simulink model "simpleSmOffPSZ"  (Simulink 7.8)
settings: Solver=FixedStepDiscrete  StartTime=0.0  StopTime=inf  FixedStep=900  RelTol=1e-3
libraries: simulink x2
settings Model: Creator=mwetter  LastModifiedBy=wbernal  ExtModeAutoUpdateStatusClock=off
settings OptimizationCC: InitFltsAndDblsToZero=on
settings DebuggingCC: SaveWithParameterizedLinksMsg=none  FcnCallInpInsideContextMsg=Use local settings  StrictBusMsg=Warning
settings SFSimCC: SimParseCustomCode=off
settings GRTTargetCC: TargetFcnLib=ansi_tfl_tmw.mat

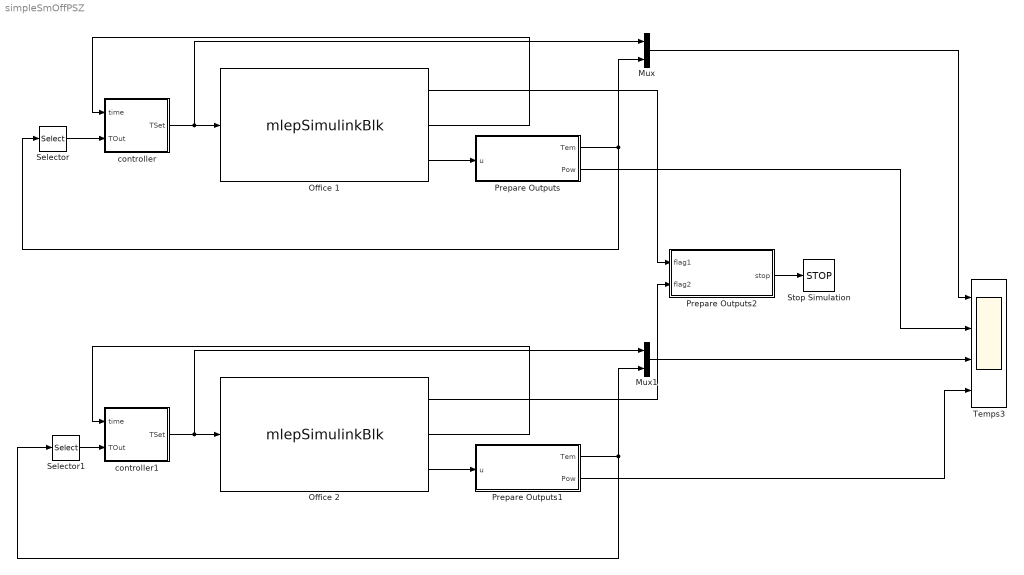
== system simpleSmOffPSZ ==
  Mux : Mux  Inputs=2
  Mux1 : Mux  Inputs=2
  Office 1 : M-S-Function  FunctionName=mlepSimulinkBlk  Parameters=progname, modelfile, weatherfile, workdir, timeout, port, host, bcvtbdir, deltaT, noutputd  mask(EnergyPlus Cosimulation){progname='C:\\EnergyPlusV8-0-0-mlep\\RunEPlus.bat', modelfile='U:\\Simulink-mlep\\SmOffPSZ1\\SmOffPSZ', weatherfile='USA_IL_Chicago-OHare.Intl.AP.725300_TMY3', workdir='U:\\Simulink-mlep\\SmOffPSZ1', timeout=2000, port=0, host='', bcvtbdir='U:\\Simulink-mlep\\bcvtb', deltaT=900, noutputd=14}
      mask prompts: progname "E+ Executable Path"; modelfile "IDF File (without extension)"; weatherfile "Weather Profile"; workdir "Working Directory"; timeout "Timeout (in milliseconds)"; port "Socket Port (0 = any available)"; host "Socket Host ('' = local host)"; bcvtbdir "BCVTB Directory"; deltaT "Time Step (in seconds)"; noutputd "Number of Real Outputs"
      mask help: This block implements cosimulation with EnergyPlus by allowing Simulink to exchange input and output data with it. Currently, EnergyPlus only supports real data.
      mask Help:
      | This block implements cosimulation with EnergyPlus by allowing Simulink to
      | exchange input and output data with it.
      | 
      | When a simulation starts, EnergyPlus is also started. It will then run in
      | parallel with Simulink. They exchange input and output data via socket
      | communication. When the simulation terminates, EnergyPlus will exit.
      | 
      | Refer to the manuals of MLE+ and/or BCVTB/EnergyPlus for details.
      | 
      | INPUTS:
      | - real: real vector input to EnergyPlus.
      | 
      | OUTPUTS:
      | - flag: status of EnergyPlus (0 if OK, if flag is non-zero, the simulation should stop).
      | - time: current simulation time of EnergyPlus, in seconds.
      | - real: real vector output from EnergyPlus.
      mask Display:
      | disp('E+\nCosimulation');
      | port_label('output', 1, 'flag');
      | port_label('output', 2, 'time');
      | port_label('output', 3, 'real');
      | % port_label('output', 4, 'int');
      | % port_label('output', 5, 'bool');
      | port_label('input', 1, 'real');
      | % port_label('input', 2, 'int');
      | % port_label('input', 3, 'bool');
      | image(imread('SmOffPSZ.png'))
  Office 2 : M-S-Function  FunctionName=mlepSimulinkBlk  Parameters=progname, modelfile, weatherfile, workdir, timeout, port, host, bcvtbdir, deltaT, noutputd  mask(EnergyPlus Cosimulation){progname='C:\\EnergyPlusV8-0-0-mlep\\RunEPlus.bat', modelfile='U:\\Simulink-mlep\\SmOffPSZ2\\SmOffPSZ', weatherfile='USA_IL_Chicago-OHare.Intl.AP.725300_TMY3', workdir='U:\\Simulink-mlep\\SmOffPSZ2', timeout=2000, port=0, host='', bcvtbdir='U:\\Simulink-mlep\\bcvtb', deltaT=900, noutputd=14}
      mask prompts: progname "E+ Executable Path"; modelfile "IDF File (without extension)"; weatherfile "Weather Profile"; workdir "Working Directory"; timeout "Timeout (in milliseconds)"; port "Socket Port (0 = any available)"; host "Socket Host ('' = local host)"; bcvtbdir "BCVTB Directory"; deltaT "Time Step (in seconds)"; noutputd "Number of Real Outputs"
      mask help: This block implements cosimulation with EnergyPlus by allowing Simulink to exchange input and output data with it. Currently, EnergyPlus only supports real data.
      mask Help:
      | This block implements cosimulation with EnergyPlus by allowing Simulink to
      | exchange input and output data with it.
      | 
      | When a simulation starts, EnergyPlus is also started. It will then run in
      | parallel with Simulink. They exchange input and output data via socket
      | communication. When the simulation terminates, EnergyPlus will exit.
      | 
      | Refer to the manuals of MLE+ and/or BCVTB/EnergyPlus for details.
      | 
      | INPUTS:
      | - real: real vector input to EnergyPlus.
      | 
      | OUTPUTS:
      | - flag: status of EnergyPlus (0 if OK, if flag is non-zero, the simulation should stop).
      | - time: current simulation time of EnergyPlus, in seconds.
      | - real: real vector output from EnergyPlus.
      mask Display:
      | disp('E+\nCosimulation');
      | port_label('output', 1, 'flag');
      | port_label('output', 2, 'time');
      | port_label('output', 3, 'real');
      | % port_label('output', 4, 'int');
      | % port_label('output', 5, 'bool');
      | port_label('input', 1, 'real');
      | % port_label('input', 2, 'int');
      | % port_label('input', 3, 'bool');
      | image(imread('SmOffPSZ.png'))
  Prepare Outputs : MATLAB Function  TreatAsAtomicUnit=on
  Prepare Outputs1 : MATLAB Function  TreatAsAtomicUnit=on
  Prepare Outputs2 : MATLAB Function  TreatAsAtomicUnit=on
  Selector : Selector  InputPortWidth=2  IndexOptions=Index vector (dialog)  Indices=[1]  OutputSizes=1
  Selector1 : Selector  InputPortWidth=2  IndexOptions=Index vector (dialog)  Indices=[1]  OutputSizes=1
  Stop Simulation : Stop
  Temps3 : Scope  NumInputPorts=4
      settings: YMin=-5~-5~-5~-5  YMax=5~5~5~5  SaveName=ScopeData3
  controller : Subsystem
  controller1 : Subsystem
  wires:
  controller/1(TSet) -> Mux/1, Office 1/1
  Office 1/2 -> controller/1(time)
  Mux/1 -> Temps3/1
  Selector/1 -> controller/2(TOut)
  Office 1/3 -> Prepare Outputs/1(u)
  Prepare Outputs/1(Tem) -> Mux/2, Selector/1
  Prepare Outputs/2(Pow) -> Temps3/2
  controller1/1(TSet) -> Mux1/1, Office 2/1
  Office 2/2 -> controller1/1(time)
  Mux1/1 -> Temps3/3
  Office 2/3 -> Prepare Outputs1/1(u)
  Prepare Outputs1/1(Tem) -> Mux1/2, Selector1/1
  Prepare Outputs1/2(Pow) -> Temps3/4
  Selector1/1 -> controller1/2(TOut)
  Prepare Outputs2/1(stop) -> Stop Simulation/1
  Office 1/1 -> Prepare Outputs2/1(flag1)
  Office 2/1 -> Prepare Outputs2/2(flag2)

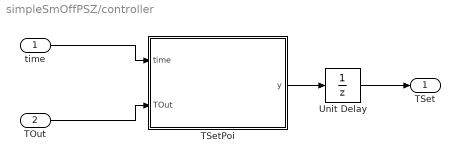
== system simpleSmOffPSZ/controller ==
  time : Inport
  TOut : Inport  Port=2
  TSetPoi : Subsystem
  Unit Delay : UnitDelay  X0=[20, 25]  SampleTime=-1
  TSet : Outport
  wires:
  time/1 -> TSetPoi/1(time)
  TOut/1 -> TSetPoi/2(TOut)
  Unit Delay/1 -> TSet/1
  TSetPoi/1(y) -> Unit Delay/1

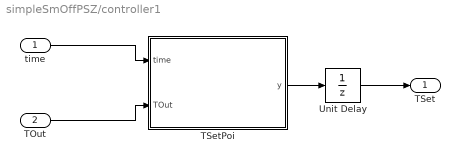
== system simpleSmOffPSZ/controller1 ==
  time : Inport
  TOut : Inport  Port=2
  TSetPoi : Subsystem
  Unit Delay : UnitDelay  X0=[20, 25]  SampleTime=-1
  TSet : Outport
  wires:
  time/1 -> TSetPoi/1(time)
  TOut/1 -> TSetPoi/2(TOut)
  Unit Delay/1 -> TSet/1
  TSetPoi/1(y) -> Unit Delay/1

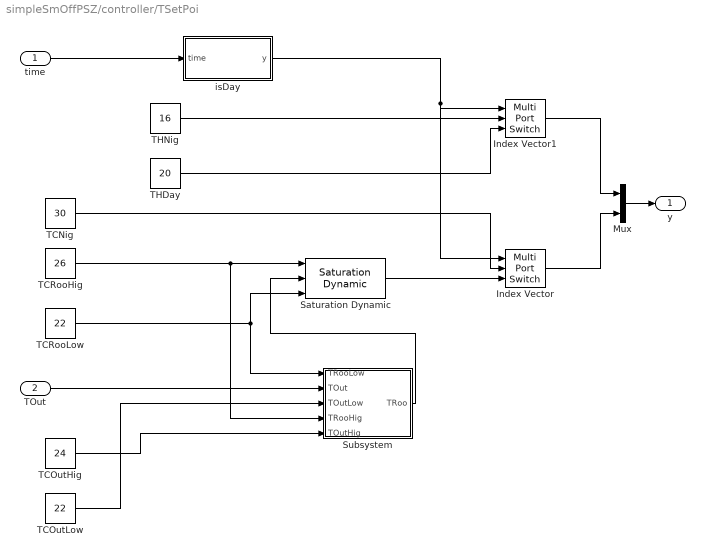
== system simpleSmOffPSZ/controller/TSetPoi ==
  time : Inport
  TOut : Inport  Port=2
  Index Vector : MultiPortSwitch  DataPortOrder=Zero-based contiguous  Inputs=2  zeroidx=on
  Index Vector1 : MultiPortSwitch  DataPortOrder=Zero-based contiguous  Inputs=2  zeroidx=on
  Mux : Mux  Inputs=2
  Saturation Dynamic : simulink/Discontinuities/Saturation Dynamic  OutMin=[]  OutMax=[]  OutDataTypeStr=Inherit: Same as second input  OutDataType=sfix(16)  OutScaling=2^-10  DoSatur=off
  Subsystem : Subsystem
  TCNig : Constant  Value=30
  TCOutHig : Constant  Value=24
  TCOutLow : Constant  Value=22
  TCRooHig : Constant  Value=26
  TCRooLow : Constant  Value=22
  THDay : Constant  Value=20
  THNig : Constant  Value=16
  isDay : Subsystem
  y : Outport
  wires:
  TOut/1 -> Subsystem/2(TOut)
  TCOutLow/1 -> Subsystem/3(TOutLow)
  TCOutHig/1 -> Subsystem/5(TOutHig)
  TCRooHig/1 -> Saturation Dynamic/1, Subsystem/4(TRooHig)
  TCRooLow/1 -> Saturation Dynamic/3, Subsystem/1(TRooLow)
  time/1 -> isDay/1(time)
  isDay/1(y) -> Index Vector/1, Index Vector1/1
  TCNig/1 -> Index Vector/2
  Subsystem/1(TRoo) -> Saturation Dynamic/2
  Saturation Dynamic/1 -> Index Vector/3
  THNig/1 -> Index Vector1/2
  THDay/1 -> Index Vector1/3
  Index Vector1/1 -> Mux/1
  Index Vector/1 -> Mux/2
  Mux/1 -> y/1

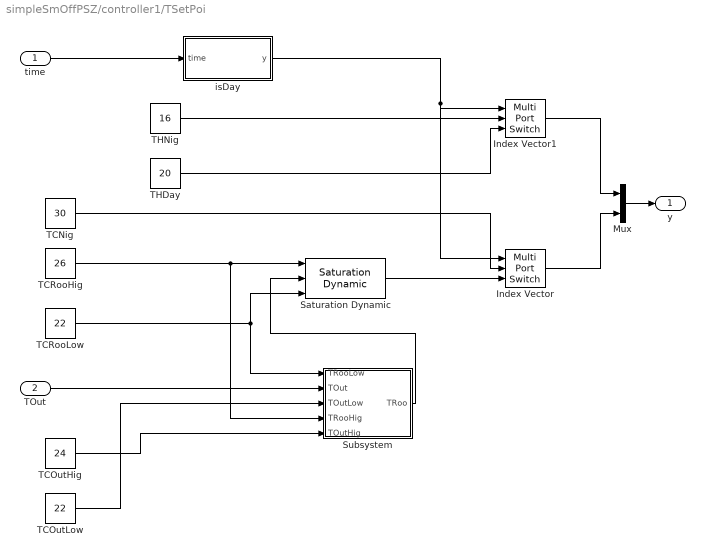
== system simpleSmOffPSZ/controller1/TSetPoi ==
  time : Inport
  TOut : Inport  Port=2
  Index Vector : MultiPortSwitch  DataPortOrder=Zero-based contiguous  Inputs=2  zeroidx=on
  Index Vector1 : MultiPortSwitch  DataPortOrder=Zero-based contiguous  Inputs=2  zeroidx=on
  Mux : Mux  Inputs=2
  Saturation Dynamic : simulink/Discontinuities/Saturation Dynamic  OutMin=[]  OutMax=[]  OutDataTypeStr=Inherit: Same as second input  OutDataType=sfix(16)  OutScaling=2^-10  DoSatur=off
  Subsystem : Subsystem
  TCNig : Constant  Value=30
  TCOutHig : Constant  Value=24
  TCOutLow : Constant  Value=22
  TCRooHig : Constant  Value=26
  TCRooLow : Constant  Value=22
  THDay : Constant  Value=20
  THNig : Constant  Value=16
  isDay : Subsystem
  y : Outport
  wires:
  TOut/1 -> Subsystem/2(TOut)
  TCOutLow/1 -> Subsystem/3(TOutLow)
  TCOutHig/1 -> Subsystem/5(TOutHig)
  TCRooHig/1 -> Saturation Dynamic/1, Subsystem/4(TRooHig)
  TCRooLow/1 -> Saturation Dynamic/3, Subsystem/1(TRooLow)
  time/1 -> isDay/1(time)
  isDay/1(y) -> Index Vector/1, Index Vector1/1
  TCNig/1 -> Index Vector/2
  Subsystem/1(TRoo) -> Saturation Dynamic/2
  Saturation Dynamic/1 -> Index Vector/3
  THNig/1 -> Index Vector1/2
  THDay/1 -> Index Vector1/3
  Index Vector1/1 -> Mux/1
  Index Vector/1 -> Mux/2
  Mux/1 -> y/1

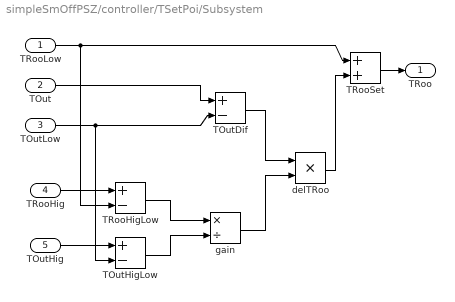
== system simpleSmOffPSZ/controller/TSetPoi/Subsystem ==
  TRooLow : Inport
  TOut : Inport  Port=2
  TOutLow : Inport  Port=3
  TRooHig : Inport  Port=4
  TOutHig : Inport  Port=5
  TOutDif : Sum  Inputs=+-
  TOutHigLow : Sum  Inputs=+-
  TRooHigLow : Sum  Inputs=+-
  TRooSet : Sum
  delTRoo : Product  RndMeth=Zero
  gain : Product  Inputs=*/
  TRoo : Outport
  wires:
  TRooHigLow/1 -> gain/1
  TOutHigLow/1 -> gain/2
  TOutDif/1 -> delTRoo/1
  gain/1 -> delTRoo/2
  delTRoo/1 -> TRooSet/2
  TRooLow/1 -> TRooSet/1, TRooHigLow/2
  TOutLow/1 -> TOutDif/2, TOutHigLow/2
  TRooHig/1 -> TRooHigLow/1
  TOutHig/1 -> TOutHigLow/1
  TRooSet/1 -> TRoo/1
  TOut/1 -> TOutDif/1

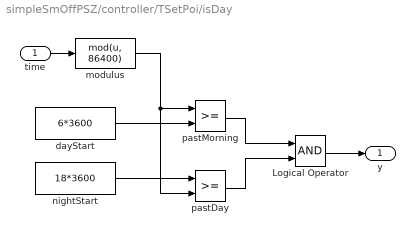
== system simpleSmOffPSZ/controller/TSetPoi/isDay ==
  time : Inport
  Logical Operator : Logic  AllPortsSameDT=off  OutDataTypeStr=boolean
  dayStart : Constant  Value=6*3600
  modulus : MATLABFcn  MATLABFcn=mod(u, 86400)
  nightStart : Constant  Value=18*3600
  pastDay : RelationalOperator  OutDataTypeStr=boolean
  pastMorning : RelationalOperator  OutDataTypeStr=boolean
  y : Outport
  wires:
  time/1 -> modulus/1
  modulus/1 -> pastMorning/1, pastDay/2
  dayStart/1 -> pastMorning/2
  nightStart/1 -> pastDay/1
  pastMorning/1 -> Logical Operator/1
  pastDay/1 -> Logical Operator/2
  Logical Operator/1 -> y/1

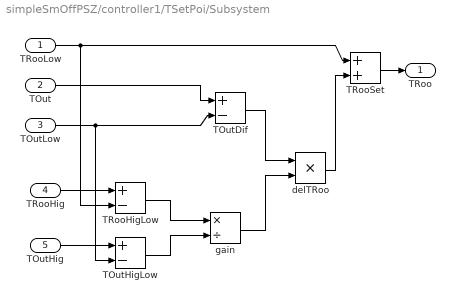
== system simpleSmOffPSZ/controller1/TSetPoi/Subsystem ==
  TRooLow : Inport
  TOut : Inport  Port=2
  TOutLow : Inport  Port=3
  TRooHig : Inport  Port=4
  TOutHig : Inport  Port=5
  TOutDif : Sum  Inputs=+-
  TOutHigLow : Sum  Inputs=+-
  TRooHigLow : Sum  Inputs=+-
  TRooSet : Sum
  delTRoo : Product  RndMeth=Zero
  gain : Product  Inputs=*/
  TRoo : Outport
  wires:
  TRooHigLow/1 -> gain/1
  TOutHigLow/1 -> gain/2
  TOutDif/1 -> delTRoo/1
  gain/1 -> delTRoo/2
  delTRoo/1 -> TRooSet/2
  TRooLow/1 -> TRooSet/1, TRooHigLow/2
  TOutLow/1 -> TOutDif/2, TOutHigLow/2
  TRooHig/1 -> TRooHigLow/1
  TOutHig/1 -> TOutHigLow/1
  TRooSet/1 -> TRoo/1
  TOut/1 -> TOutDif/1

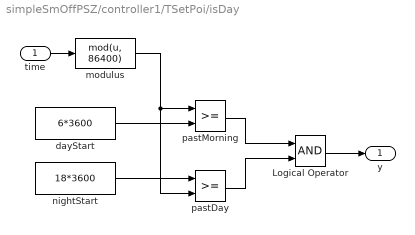
== system simpleSmOffPSZ/controller1/TSetPoi/isDay ==
  time : Inport
  Logical Operator : Logic  AllPortsSameDT=off  OutDataTypeStr=boolean
  dayStart : Constant  Value=6*3600
  modulus : MATLABFcn  MATLABFcn=mod(u, 86400)
  nightStart : Constant  Value=18*3600
  pastDay : RelationalOperator  OutDataTypeStr=boolean
  pastMorning : RelationalOperator  OutDataTypeStr=boolean
  y : Outport
  wires:
  time/1 -> modulus/1
  modulus/1 -> pastMorning/1, pastDay/2
  dayStart/1 -> pastMorning/2
  nightStart/1 -> pastDay/1
  pastMorning/1 -> Logical Operator/1
  pastDay/1 -> Logical Operator/2
  Logical Operator/1 -> y/1

== matlab function Prepare Outputs1 ==
  data: u input double; Tem output double; Pow output double
function [Tem,Pow] = fcn(u)
Pow = sum(u(3:end));
Tem = u(1:2);

== matlab function Prepare Outputs ==
  data: u input double; Tem output double; Pow output double
function [Tem,Pow] = fcn(u)
Pow = sum(u(3:end));
Tem = u(1:2);

== matlab function Prepare Outputs2 ==
  data: flag1 input double; stop output double; flag2 input double
function stop  = fcn(flag1, flag2)

if flag1 && flag2
    stop = 1;
else 
    stop = 0;
end
